simulink model "MatlabLatching"  (R2024a)
settings: Solver=VariableStepAuto  StartTime=0.0  StopTime=inf  RelTol=1e-3
libraries: simulink_extras x1, aerolibanimutils x1
settings Model: Creator=Akbar  LastModifiedBy=Akbar

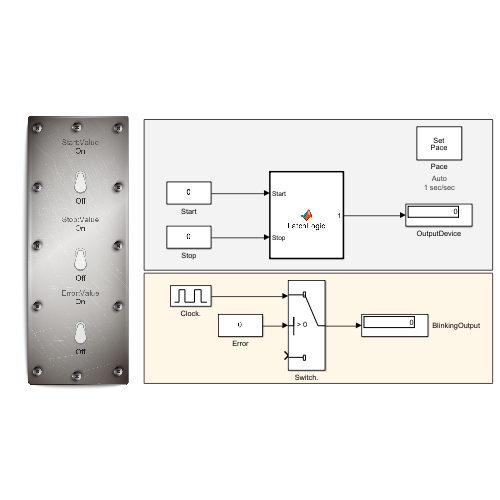
[thumbnail: Simulink's stored preview of the top-level diagram]
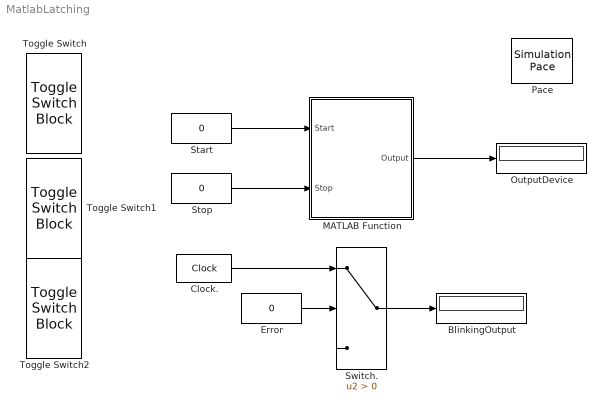
== system MatlabLatching ==
  BlinkingOutput : Display
  Clock. : simulink_extras/Flip Flops/Clock  period=2
  Error : Constant  Value=0  OutDataTypeStr=boolean
  MATLAB Function : MATLAB Function  TreatAsAtomicUnit=on
  OutputDevice : Display
  Pace : aerolibanimutils/Simulation Pace  SimulationPace=1  SleepMode=Auto  OutputPaceError=off  SampleTime=1/30
  Start : Constant  Value=0  OutDataTypeStr=boolean
  Stop : Constant  Value=0  OutDataTypeStr=boolean
  Switch. : Switch  Criteria=u2 > Threshold  SaturateOnIntegerOverflow=off  InputSameDT=off
  Toggle Switch : ToggleSwitchBlock
      settings: Values={{'Off', 'On'}, [0 1]}
  Toggle Switch1 : ToggleSwitchBlock
      settings: Values={{'Off', 'On'}, [0 1]}
  Toggle Switch2 : ToggleSwitchBlock
      settings: Values={{'Off', 'On'}, [0 1]}
  wires:
  Start/1 -> MATLAB Function/1(Start)
  Stop/1 -> MATLAB Function/2(Stop)
  MATLAB Function/1(Output) -> OutputDevice/1
  Clock./1 -> Switch./1
  Switch./1 -> BlinkingOutput/1
  Error/1 -> Switch./2

== matlab function MatlabLatching/MATLAB Function ==
  data: Start input; Output output; Stop input
function Output = LatchLogic(Start, Stop)

persistent latched;

if isempty(latched)
    latched = false; % initialize to OFF
end

% Stop has priority
if Stop
    latched = false;
elseif Start
    latched = true;
end

Output = latched;

end
